simulink model "swapna_reference1"  (R2013b)
settings: Solver=ode45  StartTime=0.0  StopTime=5  RelTol=1e-3
undefined symbols (not defined in the file): sigbuilder_block, Ts_Power
libraries: powerlib x25, powerlib_meascontrol x2
settings Model: Creator=dhamodharan  LastModifiedBy=Adroit
settings DebuggingCC: StateNameClashWarn=warning

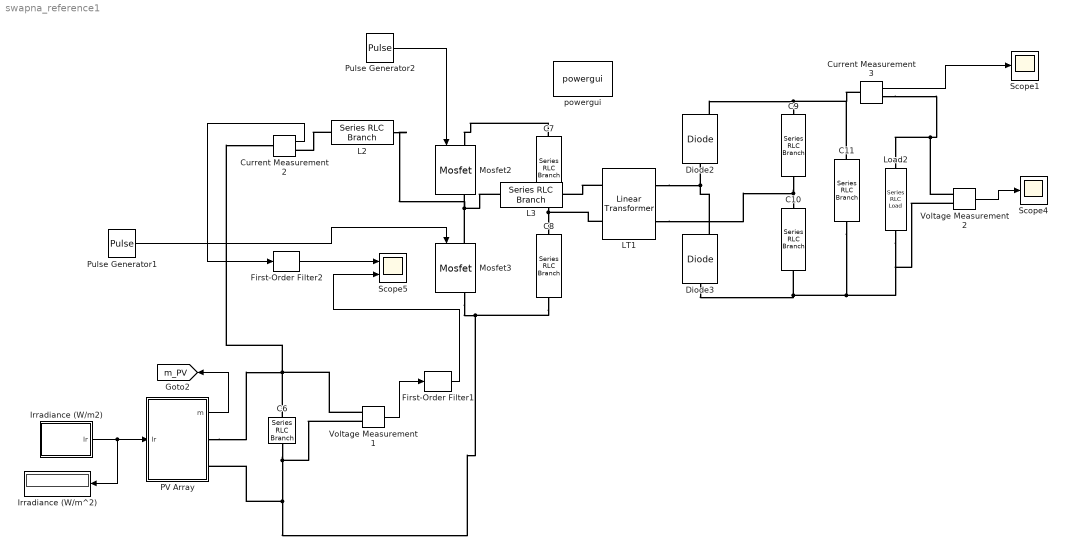
== system swapna_reference1 ==
  C10 : powerlib/Elements/Series RLC Branch  LConnTagsString=__new0  RConnTagsString=__new0  BranchType=C  Resistance=1  Inductance=1e-3  SetiL0=off  InitialCurrent=0  Capacitance=100e-9  Setx0=off  InitialVoltage=0  Measurements=None
  C11 : powerlib/Elements/Series RLC Branch  LConnTagsString=__new0  RConnTagsString=__new0  BranchType=C  Resistance=1  Inductance=1e-3  SetiL0=off  InitialCurrent=0  Capacitance=2000e-6  Setx0=off  InitialVoltage=0  Measurements=None
  C6 : powerlib/Elements/Series RLC Branch  LConnTagsString=__new0  RConnTagsString=__new0  BranchType=C  Resistance=1.0  Inductance=1.0  SetiL0=off  InitialCurrent=0  Capacitance=1000e-6  Setx0=off  InitialVoltage=0  Measurements=Branch voltage
  C7 : powerlib/Elements/Series RLC Branch  LConnTagsString=__new0  RConnTagsString=__new0  BranchType=C  Resistance=1  Inductance=1e-3  SetiL0=off  InitialCurrent=0  Capacitance=10e-6  Setx0=off  InitialVoltage=0  Measurements=None
  C8 : powerlib/Elements/Series RLC Branch  LConnTagsString=__new0  RConnTagsString=__new0  BranchType=C  Resistance=1  Inductance=1e-3  SetiL0=off  InitialCurrent=0  Capacitance=10e-6  Setx0=off  InitialVoltage=0  Measurements=None
  C9 : powerlib/Elements/Series RLC Branch  LConnTagsString=__new0  RConnTagsString=__new0  BranchType=C  Resistance=1  Inductance=1e-3  SetiL0=off  InitialCurrent=0  Capacitance=100e-9  Setx0=off  InitialVoltage=0  Measurements=None
  Current Measurement2 : powerlib/Measurements/Current Measurement  PhasorSimulation=off  OutputType=Complex  PSBequivalent=0
  Current Measurement3 : powerlib/Measurements/Current Measurement  PhasorSimulation=off  OutputType=Complex  PSBequivalent=0
  Diode2 : powerlib/Power Electronics/Diode  Ron=0.001  Lon=0  Vf=0.8  IC=0  UseSnubber=off  Rs=500  Cs=250e-9  Measurements=on
  Diode3 : powerlib/Power Electronics/Diode  Ron=0.001  Lon=0  Vf=0.8  IC=0  UseSnubber=off  Rs=500  Cs=250e-9  Measurements=on
  First-Order Filter1 : powerlib_meascontrol/Filters/First-Order Filter  FilterType=Lowpass  Tc=1/10  Ts=0  Initialize=on  Vac_Init=[0, 0, 50]  Vdc_Init=0  PlotResponse=off  FreqRange="[0,  200,  1]"
  First-Order Filter2 : powerlib_meascontrol/Filters/First-Order Filter  FilterType=Lowpass  Tc=1/1  Ts=0  Initialize=on  Vac_Init=[0, 0, 50]  Vdc_Init=0  PlotResponse=off  FreqRange="[0,  200,  1]"
  "Irradiance (W/m2) " : Subsystem  Tag=STV Subsys  LoadFcn=sigbuilder_block('load');  StartFcn=sigbuilder_block('start');  StopFcn=sigbuilder_block('stop');  ClipboardFcn=sigbuilder_block('clipboard');  mask(Sigbuilder block){}
      mask help: Sigbuilder GUI
      mask init:
      | if ~strcmp(get_param(bdroot(gcbh),'SimulationStatus'),'stopped') tuvar = sigbuilder_block('maskInit'); end
      settings: CopyFcn=sigbuilder_block('copy');  DeleteFcn=sigbuilder_block('delete');  ModelCloseFcn=sigbuilder_block('modelClose');  PreSaveFcn=sigbuilder_block('preSave');  PauseFcn=sigbuilder_block('pause')  ContinueFcn=sigbuilder_block('continue')  NameChangeFcn=sigbuilder_block('namechange');  OpenFcn=sigbuilder_block('open',[6.75 6 954 505.5 ]);  CloseFcn=sigbuilder_block('close');
      mask Display: plot(0,0,100,100,[10,10,40,40,10],[80,20,20,80,80],[40,10],[50,50], [40,27,10],[65,72,56],[40,25,25,10],[28,28,43,43]);
  Irradiance (W/m^2) : Display
      settings: Format=bank  Decimation=1000
  L2 : powerlib/Elements/Series RLC Branch  LConnTagsString=__new0  RConnTagsString=__new0  BranchType=L  Resistance=1  Inductance=100e-6  SetiL0=off  InitialCurrent=0  Capacitance=1e-6  Setx0=off  InitialVoltage=0  Measurements=None
  L3 : powerlib/Elements/Series RLC Branch  LConnTagsString=__new0  RConnTagsString=__new0  BranchType=L  Resistance=1  Inductance=0.001e-6  SetiL0=off  InitialCurrent=0  Capacitance=1e-6  Setx0=off  InitialVoltage=0  Measurements=None
  LT1 : powerlib/Elements/Linear Transformer  UNITS=pu  NominalPower=[ 200 66.66e3 ]  winding1="[ 20 0.002  0.08 ]"  winding2="[ 200 0.002  0.08 ]"  ThreeWindings=off  winding3=[ 315e3 0.002 0.08 ]  RmLm=[0.2 0.2 ]  Measurements=None  DataType=off
  Load2 : powerlib/Elements/Series RLC Load  LConnTagsString=a  RConnTagsString=__new0  NominalVoltage=120  NominalFrequency=66e3  ActivePower=30  InductivePower=0  CapacitivePower=0  Setx0=off  InitialVoltage=0  SetiL0=off  InitialCurrent=0  Measurements=None
  Mosfet2 : powerlib/Power Electronics/Mosfet  Ron=0.1  Lon=0  Rd=0.01  Vfd=0  IC=0  Rs=1e5  Cs=inf  Measurements=on
  Mosfet3 : powerlib/Power Electronics/Mosfet  Ron=0.1  Lon=0  Rd=0.01  Vfd=0  IC=0  Rs=1e5  Cs=inf  Measurements=on
  PV Array : Subsystem  mask(PV array){ModuleType=Kyocera KD135GX-LP, Ncell=36, Nser=1, Npar=2, ModuleParameters=[ 22.0999  8.36955  17.7  7.62959 ], ModelParameters=[ 0.10593  142.84  2.6762e-06  8.3758  1.5 ], Ts=Ts_Power, PlotVI_module=off, PlotVI_array=off}
      mask prompts: ModuleType "Module type:"; Ncell "Number of cells per module"; Nser "Number of series-connected  modules per string"; Npar "Number of parallel strings"; ModuleParameters "Module specifications under STC  [  Voc, Isc, Vmp, Imp ]"; ModelParameters "Model parameters for 1 module [ Rs, Rp, Isat, Iph, Qd ]"; Ts "Sample time"; PlotVI_module "Display  I-V and  P-V characteritics of one module"; PlotVI_array "Display  I-V and  P-V characteritics of array"
      mask help:
      | Model a PV array
      |
      | PV array consists of Npar strings of modules connected in parallel, each string consisting of Nser modules connected in series.
      |
      | The four PV model parameters (photo-generated current Iph, diode saturation current Isat, parallel resistance Rp and  series resistance Rs) are adjuted to fit the following four module characteristics measured under standard test conditions (STC : irradiance 1000 W/m^2, cell temperature=25 deg. C) and assuming a given "diode quality factor" (Qd) for the semiconductor:
      |   Voc = open circuit voltage
      |   Isc = short-circuit current
      |   Vmp,Imp = voltage and current at maximum power point
      |
      | Select a 'Module type' and then press Apply to see module parameters.
      | Note: Module characteristics are extracted from NREL System Advisor Model.
      mask init:
      | BlockName=gcb;
      | 
      | % Solar Modules Specifications
      | %=============================
      | %
      | Type=1;
      | SolarModuleSpec(Type).Desc= 'Kyocera KD135GX-LP';
      | SolarModuleSpec(Type).nCells= 36;              % Number of cells in series
      | SolarModuleSpec(Type).Pmp= 135.044;            % Maximum power (W)
      | SolarModuleSpec(Type).Vmp= 17.7;               % Maximum power voltage (V) 
      | SolarModuleSpec(Type).Imp= 7.62959;            % Maximum power current (A)
      | SolarModuleSpec(Type).Voc= 22.0999;            % Open circuit voltage (V)
      | SolarModuleSpec(Type).Isc= 8.36955;            % Short circuit current (A)
      | SolarModuleSpec(Type).TempC_Pmp= -6.445e-001;  % Maximum power temp. coefficient (W/deg.C)
      | SolarModuleSpec(Type).TempC_Vmp= -8.200e-002;  % Maximum power voltage temp. coefficient (V/deg.C)
      | SolarModuleSpec(Type).TempC_Imp= -1.068e-003;  % Maximum power current temp. coefficient (A/deg.C
      | SolarModuleSpec(Type).TempC_Voc= -8.000e-002;  % Open circuit voltage temp. coefficient (V/deg.C)
      | SolarModuleSpec(Type).TempC_Isc= 5.022e-003;   % Short circuit current temp. coefficient (A/deg.C)
      | SolarModuleSpec(Type).Rs= 0.10593;             % Series resistance of PV model (ohms)
      | SolarModuleSpec(Type).Rp= 142.84;              % Parallel resistance of PV model (ohms)
      | SolarModuleSpec(Type).Isat= 2.6762e-006;       % Diode saturation current of PV model (A)
      | SolarModuleSpec(Type).Iph=  8.3758;            % Light-generated photo-current  of PV model (A)
      | SolarModuleSpec(Type).Qd= 1.5;                 % Diode quality factor of PV model
      | %-------------------------------------------------------------------------
      | %
      | Type=2;
      | SolarModuleSpec(Type).Desc= 'Kyocera KD205GX-LP';
      | SolarModuleSpec(Type).nCells= 54;              % Number of cells in series
      | SolarModuleSpec(Type).Pmp= 205.075;            % Maximum power (W)
      | SolarModuleSpec(Type).Vmp= 26.6;               % Maximum power voltage (V) 
      | SolarModuleSpec(Type).Imp= 7.70959;            % Maximum power current (A)
      | SolarModuleSpec(Type).Voc= 33.1999;            % Open circuit voltage (V)
      | SolarModuleSpec(Type).Isc= 8.35955;            % Short circuit current (A)
      | SolarModuleSpec(Type).TempC_Pmp= -9.770e-001;  % Maximum power temp. coefficient (W/deg.C)
      | SolarModuleSpec(Type).TempC_Vmp= -1.230e-001;  % Maximum power voltage temp. coefficient (V/deg.C)
      | SolarModuleSpec(Type).TempC_Imp= -1.079e-003;  % Maximum power current temp. coefficient (A/deg.C
      | SolarModuleSpec(Type).TempC_Voc= -1.200e-001;  % Open circuit voltage temp. coefficient (V/deg.C)
      | SolarModuleSpec(Type).TempC_Isc= 5.016e-003;   % Short circuit current temp. coefficient (A/deg.C)
      | SolarModuleSpec(Type).Rs= 0.15943;             % Series resistance of PV model (ohms)
      | SolarModuleSpec(Type).Rp= 931.61;              % Parallel resistance of PV model (ohms)
      | SolarModuleSpec(Type).Isat= 2.647e-006;        % Diode saturation current of PV model (A)
      | SolarModuleSpec(Type).Iph= 8.3652;             % Light-generated photo-current  of PV model (A)
      | SolarModuleSpec(Type).Qd= 1.5;                 % Diode quality factor of PV model
      | %-------------------------------------------------------------------------
      | %
      | Type=3;
      | SolarModuleSpec(Type).Desc= 'Mitsubishi PV-UD190MF5';
      | SolarModuleSpec(Type).nCells= 50;              % Number of cells in series
      | SolarModuleSpec(Type).Pmp= 190.503;            % Maximum power (W)
      | SolarModuleSpec(Type).Vmp= 24.6999;            % Maximum power voltage (V) 
      | SolarModuleSpec(Type).Imp= 7.71272;            % Maximum power current (A)
      | SolarModuleSpec(Type).Voc= 30.8006;            % Open circuit voltage (V)
      | SolarModuleSpec(Type).Isc= 8.23289;            % Short circuit current (A)
      | SolarModuleSpec(Type).TempC_Pmp= -8.597e-001;  % Maximum power temp. coefficient (W/deg.C)
      | SolarModuleSpec(Type).TempC_Vmp= -1.090e-001;  % Maximum power voltage temp. coefficient (V/deg.C)
      | SolarModuleSpec(Type).TempC_Imp= -7.713e-004;  % Maximum power current temp. coefficient (A/deg.C
      | SolarModuleSpec(Type).TempC_Voc= -1.050e-001;  % Open circuit voltage temp. coefficient (V/deg.C)
      | SolarModuleSpec(Type).TempC_Isc= 4.446e-003;   % Short circuit current temp. coefficient (A/deg.C)
      | SolarModuleSpec(Type).Rs= 0.14743;             % Series resistance of PV model (ohms)
      | SolarModuleSpec(Type).Rp= 1982.4;              % Parallel resistance of PV model (ohms)
      | SolarModuleSpec(Type).Isat= 2.5519e-006;       % Diode saturation current of PV model (A)
      | SolarModuleSpec(Type).Iph= 8.2998;             % Light-generated photo-current  of PV model (A)
      | SolarModuleSpec(Type).Qd= 1.5;                 % Diode quality factor of PV model
      | %-------------------------------------------------------------------------
      | %
      | Type=4;
      | SolarModuleSpec(Type).Desc= 'Sanyo HIP-225HDE1';
      | SolarModuleSpec(Type).nCells= 60;              % Number of cells in series
      | SolarModuleSpec(Type).Pmp= 224.899;            % Maximum power (W)
      | SolarModuleSpec(Type).Vmp= 33.9;               % Maximum power voltage (V) 
      | SolarModuleSpec(Type).Imp= 6.63419;            % Maximum power current (A)
      | SolarModuleSpec(Type).Voc= 41.7984;            % Open circuit voltage (V)
      | SolarModuleSpec(Type).Isc= 7.13383;            % Short circuit current (A)
      | SolarModuleSpec(Type).TempC_Pmp= -6.925e-001;  % Maximum power temp. coefficient (W/deg.C)
      | SolarModuleSpec(Type).TempC_Vmp= -1.010e-001;  % Maximum power voltage temp. coefficient (V/deg.C)
      | SolarModuleSpec(Type).TempC_Imp= -6.634e-004;  % Maximum power current temp. coefficient (A/deg.C
      | SolarModuleSpec(Type).TempC_Voc= -1.050e-001;  % Open circuit voltage temp. coefficient (V/deg.C)
      | SolarModuleSpec(Type).TempC_Isc= 2.140e-003;   % Short circuit current temp. coefficient (A/deg.C)
      | SolarModuleSpec(Type).Rs=  0.24713;            % Series resistance of PV model (ohms)
      | SolarModuleSpec(Type).Rp= 1215.2;              % Parallel resistance of PV model (ohms)
      | SolarModuleSpec(Type).Isat= 2.697e-007;        % Diode saturation current of PV model (A)
      | SolarModuleSpec(Type).Iph= 7.1361;             % Light-generated photo-current  of PV model (A)
      | SolarModuleSpec(Type).Qd= 1.5;                 % Diode quality factor of PV model
      | %-------------------------------------------------------------------------
      | %
      | Type=5;
      | % SolarModuleSpec(Type).Desc= 'SunPower SPR-305-WHT [2009]';
      | % SolarModuleSpec(Type).nCells= 96;              % Number of cells in series
      | % SolarModuleSpec(Type).Pmp= 304.248;            % Maximum power (W)
      | % SolarModuleSpec(Type).Vmp= 54.4299;            % Maximum power voltage (V) 
      | % SolarModuleSpec(Type).Imp= 5.58972;            % Maximum power current (A)
      | % SolarModuleSpec(Type).Voc= 65.3099;            % Open circuit voltage (V)
      | % SolarModuleSpec(Type).Isc= 5.9197;             % Short circuit current (A)
      | % SolarModuleSpec(Type).TempC_Pmp= -1.229e+000;  % Maximum power temp. coefficient (W/deg.C)
      | % SolarModuleSpec(Type).TempC_Vmp= -2.030e-001;  % Maximum power voltage temp. coefficient (V/deg.C)
      | % SolarModuleSpec(Type).TempC_Imp= -1.733e-003;  % Maximum power current temp. coefficient (A/deg.C
      | % SolarModuleSpec(Type).TempC_Voc= -1.930e-001;  % Open circuit voltage temp. coefficient (V/deg.C)
      | % SolarModuleSpec(Type).TempC_Isc= 2.368e-003;   % Short circuit current temp. coefficient (A/deg.C)
      | 
      | %NREL : 2007(E)
      | SolarModuleSpec(Type).Desc= 'SunPower SPR-305-WHT';
      | SolarModuleSpec(Type).nCells= 96;              % Number of cells in series
      | SolarModuleSpec(Type).Pmp= 305.2;              % Maximum power (W)
      | SolarModuleSpec(Type).Vmp= 54.70;              % Maximum power voltage (V) 
      | SolarModuleSpec(Type).Imp= 5.58;               % Maximum power current (A)
      | SolarModuleSpec(Type).Voc= 64.20;              % Open circuit voltage (V)
      | SolarModuleSpec(Type).Isc= 5.96;               % Short circuit current (A)
      | SolarModuleSpec(Type).TempC_Pmp= -1.154e+000;  % Maximum power temp. coefficient (W/deg.C)
      | SolarModuleSpec(Type).TempC_Vmp= -1.860e-001;  % Maximum power voltage temp. coefficient (V/deg.C)
      | SolarModuleSpec(Type).TempC_Imp= -2.120e-003;  % Maximum power current temp. coefficient (A/deg.C
      | SolarModuleSpec(Type).TempC_Voc= -1.770e-001;  % Open circuit voltage temp. coefficient (V/deg.C)
      | SolarModuleSpec(Type).TempC_Isc= 3.516e-003;   % Short circuit current temp. coefficient (A/deg.C)
      | SolarModuleSpec(Type).Rs= 0.0380;              % Series resistance of PV model (ohms)
      | SolarModuleSpec(Type).Rp= 993.5;               % Parallel resistance of PV model (ohms)
      | SolarModuleSpec(Type).Isat= 3.1949e-8;         % Diode saturation current of PV model (A)
      | SolarModuleSpec(Type).Iph= 5.9602;             % Light-generated photo-current  of PV model (A)
      | SolarModuleSpec(Type).Qd= 1.3;                 % Diode quality factor of PV model
      | %-------------------------------------------------------------------------
      | %
      | Type=6;
      | SolarModuleSpec(Type).Desc= 'Suntech STP270S-24_Vb';
      | SolarModuleSpec(Type).nCells= 72;              % Number of cells in series
      | SolarModuleSpec(Type).Pmp= 269.843;            % Maximum power (W)
      | SolarModuleSpec(Type).Vmp= 35;                 % Maximum power voltage (V) 
      | SolarModuleSpec(Type).Imp= 7.70979;            % Maximum power current (A)
      | SolarModuleSpec(Type).Voc= 44.4999;            % Open circuit voltage (V)
      | SolarModuleSpec(Type).Isc= 8.19978;            % Short circuit current (A)
      | SolarModuleSpec(Type).TempC_Pmp= -1.204e+000;  % Maximum power temp. coefficient (W/deg.C)
      | SolarModuleSpec(Type).TempC_Vmp= -1.567e-001;  % Maximum power voltage temp. coefficient (V/deg.C)
      | SolarModuleSpec(Type).TempC_Imp= 1.234e-004;   % Maximum power current temp. coefficient (A/deg.C
      | SolarModuleSpec(Type).TempC_Voc= -1.504e-001;  % Open circuit voltage temp. coefficient (V/deg.C)
      | SolarModuleSpec(Type).TempC_Isc= 4.969e-003;   % Short circuit current temp. coefficient (A/deg.C)
      | SolarModuleSpec(Type).Rs= 0.32042;             % Series resistance of PV model (ohms)
      | SolarModuleSpec(Type).Rp= 3363.6;              % Parallel resistance of PV model (ohms)
      | SolarModuleSpec(Type).Isat= 2.419e-006;        % Diode saturation current of PV model (A)
      | SolarModuleSpec(Type).Iph= 8.2934;             % Light-generated photo-current  of PV model (A)
      | SolarModuleSpec(Type).Qd= 1.5;                 % Diode quality factor of PV model
      | % 
      | %-------------------------------------------------------------------------
      | %
      | Type=7;
      | SolarModuleSpec(Type).Desc= 'Canadian Solar CS5P-220M';
      | SolarModuleSpec(Type).nCells= 96;              % Number of cells in series
      | SolarModuleSpec(Type).Pmp= 219.72;             % Maximum power (W)
      | SolarModuleSpec(Type).Vmp= 48.3159;            % Maximum power voltage (V) 
      | SolarModuleSpec(Type).Imp= 4.54758;            % Maximum power current (A)
      | SolarModuleSpec(Type).Voc= 59.2618;            % Open circuit voltage (V)
      | SolarModuleSpec(Type).Isc= 5.09261;            % Short circuit current (A)
      | SolarModuleSpec(Type).TempC_Pmp= -1.031e+000;  % Maximum power temp. coefficient (W/deg.C)
      | SolarModuleSpec(Type).TempC_Vmp= -2.355e-001;  % Maximum power voltage temp. coefficient (V/deg.C)
      | SolarModuleSpec(Type).TempC_Imp= 8.231e-004;   % Maximum power current temp. coefficient (A/deg.C
      | SolarModuleSpec(Type).TempC_Voc= -2.170e-001;  % Open circuit voltage temp. coefficient (V/deg.C)
      | SolarModuleSpec(Type).TempC_Isc= 2.022e-003;   % Short circuit current temp. coefficient (A/deg.C)
      | SolarModuleSpec(Type).Rs= 0.24806;             % Series resistance of PV model (ohms)
      | SolarModuleSpec(Type).Rp= 235.76;              % Parallel resistance of PV model (ohms)
      | SolarModuleSpec(Type).Isat= 1.4435e-006;       % Diode saturation current of PV model (A)
      | SolarModuleSpec(Type).Iph= 5.098;              % Light-generated photo-current  of PV model (A)
      | SolarModuleSpec(Type).Qd= 1.5;                 % Diode quality factor of PV model
      | %-------------------------------------------------------------------------
      | %
      | Type=8;
      | SolarModuleSpec(Type).Desc= 'BP Solar SX3190';
      | SolarModuleSpec(Type).nCells= 50;              % Number of cells in series
      | SolarModuleSpec(Type).Pmp= 190.258;            % Maximum power (W)
      | SolarModuleSpec(Type).Vmp= 24.3003;            % Maximum power voltage (V) 
      | SolarModuleSpec(Type).Imp= 7.82945;            % Maximum power current (A)
      | SolarModuleSpec(Type).Voc= 30.6021;            % Open circuit voltage (V)
      | SolarModuleSpec(Type).Isc= 8.51029;            % Short circuit current (A)
      | SolarModuleSpec(Type).TempC_Pmp= -9.306e-001;  % Maximum power temp. coefficient (W/deg.C)
      | SolarModuleSpec(Type).TempC_Vmp= -1.140e-001;  % Maximum power voltage temp. coefficient (V/deg.C)
      | SolarModuleSpec(Type).TempC_Imp= -1.566e-003;  % Maximum power current temp. coefficient (A/deg.C
      | SolarModuleSpec(Type).TempC_Voc= -1.110e-001;  % Open circuit voltage temp. coefficient (V/deg.C)
      | SolarModuleSpec(Type).TempC_Isc= 5.532e-003;   % Short circuit current temp. coefficient (A/deg.C)
      | SolarModuleSpec(Type).Rs= 0.17514;             % Series resistance of PV model (ohms)
      | SolarModuleSpec(Type).Rp= 766.69;              % Parallel resistance of PV model (ohms)
      | SolarModuleSpec(Type).Isat= 2.8943e-006;       % Diode saturation current of PV model (A)
      | SolarModuleSpec(Type).Iph= 8.5156;             % Light-generated photo-current  of PV model (A)
      | SolarModuleSpec(Type).Qd= 1.5;                 % Diode quality factor of PV model
      | %-------------------------------------------------------------------------
      | %
      | Type=9;
      | SolarModuleSpec(Type).Desc= 'First Solar FS-272';
      | SolarModuleSpec(Type).nCells= 116;             % Number of cells in series
      | SolarModuleSpec(Type).Pmp= 71.326;             % Maximum power (W)
      | SolarModuleSpec(Type).Vmp= 70.558;             % Maximum power voltage (V) 
      | SolarModuleSpec(Type).Imp= 1.01088;            % Maximum power current (A)
      | SolarModuleSpec(Type).Voc= 94.5738;            % Open circuit voltage (V)
      | SolarModuleSpec(Type).Isc= 1.18103;            % Short circuit current (A)
      | SolarModuleSpec(Type).TempC_Pmp= -2.332e-001;  % Maximum power temp. coefficient (W/deg.C)
      | SolarModuleSpec(Type).TempC_Vmp= -2.060e-001;  % Maximum power voltage temp. coefficient (V/deg.C)
      | SolarModuleSpec(Type).TempC_Imp= -3.538e-004;  % Maximum power current temp. coefficient (A/deg.C
      | SolarModuleSpec(Type).TempC_Voc= -2.690e-001;  % Open circuit voltage temp. coefficient (V/deg.C)
      | SolarModuleSpec(Type).TempC_Isc= 5.433e-004;   % Short circuit current temp. coefficient (A/deg.C)
      | SolarModuleSpec(Type).Rs= 9.1791;              % Series resistance of PV model (ohms)
      | SolarModuleSpec(Type).Rp= 877.05;              % Parallel resistance of PV model (ohms)
      | SolarModuleSpec(Type).Isat= 3.7627e-007;       % Diode saturation current of PV model (A)
      | SolarModuleSpec(Type).Iph= 1.1934;             % Light-generated photo-current  of PV model (A)
      | SolarModuleSpec(Type).Qd= 2.0;                 % Diode quality factor of PV model
      | %-------------------------------------------------------------------------
      | %
      | Type=10;
      | SolarModuleSpec(Type).Desc= 'SunPower 128-cell Module';
      | SolarModuleSpec(Type).nCells= 128;             % Number of cells in series
      | SolarModuleSpec(Type).Pmp= 400.048;            % Maximum power (W)
      | SolarModuleSpec(Type).Vmp= 72.8992;            % Maximum power voltage (V) 
      | SolarModuleSpec(Type).Imp= 5.48769;            % Maximum power current (A)
      | SolarModuleSpec(Type).Voc= 85.2983;            % Open circuit voltage (V)
      | SolarModuleSpec(Type).Isc= 5.8675;             % Short circuit current (A)
      | SolarModuleSpec(Type).TempC_Pmp= -1.638e+000;  % Maximum power temp. coefficient (W/deg.C)
      | SolarModuleSpec(Type).TempC_Vmp= -2.760e-001;  % Maximum power voltage temp. coefficient (V/deg.C)
      | SolarModuleSpec(Type).TempC_Imp= -1.690e-003;  % Maximum power current temp. coefficient (A/deg.C
      | SolarModuleSpec(Type).TempC_Voc= -2.664e-001;  % Open circuit voltage temp. coefficient (V/deg.C)
      | SolarModuleSpec(Type).TempC_Isc= 1.837e-003;   % Short circuit current temp. coefficient (A/deg.C)
      | SolarModuleSpec(Type).Rs= 0.12264;             % Series resistance of PV model (ohms)
      | SolarModuleSpec(Type).Rp= 859.93;              % Parallel resistance of PV model (ohms)
      | SolarModuleSpec(Type).Isat= 6.3567e-009;       % Diode saturation current of PV model (A)
      | SolarModuleSpec(Type).Iph= 5.8683;             % Light-generated photo-current  of PV model (A)
      | SolarModuleSpec(Type).Qd= 1.2;                 % Diode quality factor of PV model
      | %-------------------------------------------------------------------------
      | 
      | Type=strmatch(ModuleType,char(SolarModuleSpec.Desc));
      | 
      | k= 1.3806e-23; % Boltman consstant (J.K^-1)
      | q=1.6022e-19;  % electron charge  (C)
      | T=273+25;
      | 
      | nCells=SolarModuleSpec(Type).nCells;
      | Voc=SolarModuleSpec(Type).Voc;
      | Isc=SolarModuleSpec(Type).Isc;
      | Vm=SolarModuleSpec(Type).Vmp;
      | Im=SolarModuleSpec(Type).Imp;
      | 
      | set_param(BlockName,'Ncell',num2str(nCells));
      | str=sprintf('[ %g  %g  %g  %g ]',Voc,Isc,Vm,Im);
      | set_param(BlockName,'ModuleParameters',str);
      | 
      | Rs=SolarModuleSpec(Type).Rs;
      | Rp=SolarModuleSpec(Type).Rp; 
      | Isat=SolarModuleSpec(Type).Isat;
      | Iph=SolarModuleSpec(Type).Iph;            
      | Qd=SolarModuleSpec(Type).Qd;
      | 
      | VT=k*T/q*nCells*Qd;
      | 
      | str=sprintf('[ %g  %g  %g  %g  %g ]',Rs,Rp,Isat,Iph, Qd);
      | set_param(BlockName,'ModelParameters',str)
      | 
      | Iph_array=Iph*Npar;
      | Isat_array=Isat*Npar;
      | VT_array=VT*Nser;
      | Rs_array=Rs*Nser/Npar;
      | Rp_array=Rp*Nser/Npar;
      | %
      | %% Plot I-V & P-V characteristics of one module
      | %==============================================
      | if PlotVI_module | PlotVI_array
      |     assignin('base','Voc',Voc);
      |     assignin('base','Isc',Isc);
      |     assignin('base','Rs',Rs);
      |     assignin('base','Rp',Rp);
      |     assignin('base','Isat',Isat);
      |     assignin('base','VT',VT);
      |      
      |     if PlotVI_module, 
      |         F1=figure('Name','I-V and P-V characteristics of one module at 25 deg.C');
      |     end
      |     if PlotVI_array ,
      |         F2=figure('Name','I-V and P-V characteristics of array at 25 deg.C');  
      |     end
      |     load_system('PV_model_Param');
      |     
      |     for ksun=1:-0.25:0.25
      |         assignin('base','Iph',Iph*ksun)
      |         sim('PV_model_Param');
      |         n=find(I_PV>=0);
      |         I_PV=I_PV(n);
      |         V_PV=V_PV(n);
      |         P_PV=V_PV.*I_PV;
      |         
      |         if PlotVI_module
      |             figure(F1);
      |             subplot(211)
      |             if ksun==1
      |                 plot(V_PV,I_PV,'b',[0  Vm Voc], [Isc Im 0],'ro')
      |                 text(Voc/15,Isc*1.1,'1 kW/m^2')
      |                 hold on
      |                 grid
      |             else
      |                 plot(V_PV,I_PV,'--m')
      |                 text(Voc/15, Isc*(ksun+0.1) , sprintf('%g kW/m^2',ksun))
      |             end
      | 
      |             subplot(212) 
      |             if ksun==1
      |                 plot(V_PV,P_PV,'b',[0  Vm Voc], [0 Im*Vm 0],'ro')
      |                 text(Vm*1.02,Vm*Im,'1 kW/m^2')
      |                 hold on
      |                 grid
      |             else
      |                 n= find(P_PV==max(P_PV));
      |                 plot(V_PV,P_PV,'--m', V_PV(n) , P_PV(n),'mo')
      |                 text(Vm*1.02, Vm*Im*ksun, sprintf('%g kW/m^2',ksun))
      |             end
      |             subplot(211)
      |             ylabel('Current (A)')
      |             xlabel('Voltage (V)')
      |             title(sprintf('Module type: %s',SolarModuleSpec(Type).Desc))
      |             axis_xy=axis;
      |             axis_xy(4)=Isc*1.2;
      |             axis(axis_xy);
      |             
      |             subplot(212)
      |             ylabel('Power (W)')
      |             xlabel('Voltage (V)')
      |             axis_xy=axis;
      |             axis_xy(4)=Vm*Im*1.2;
      |             axis(axis_xy);
      |                   
      |             set_param(BlockName,'PlotVI_module', 'off')
      |         end
      |         
      |         if PlotVI_array
      |             figure(F2);
      |             subplot(211)
      |             if ksun==1
      |                 plot(V_PV*Nser,I_PV*Npar,'b',[0  Vm Voc]*Nser, [Isc Im 0]*Npar,'ro')
      |                 text(Voc/15*Nser,Isc*1.1*Npar,'1 kW/m^2')
      |                 hold on
      |                 grid
      |             else
      |                 plot(V_PV*Nser,I_PV*Npar,'--m')
      |                 text(Voc*Nser/15, Isc*Npar*(ksun+0.1) , sprintf('%g kW/m^2',ksun))
      |             end
      |            
      | 
      |             subplot(212)
      |             if ksun==1
      |                 plot(V_PV*Nser,P_PV*Nser*Npar,'b',[0  Vm Voc]*Nser, [0 Im*Vm 0]*Nser*Npar,'ro')
      |                 text(Vm*Nser*1.02,Vm*Im*Nser*Npar,'1 kW/m^2')
      |                 hold on
      |                 grid
      |             else
      |                 n= find(P_PV==max(P_PV));
      |                 plot(V_PV*Nser,P_PV*Nser*Npar,'--m', V_PV(n)*Nser , P_PV(n)*Nser*Npar,'mo')
      |                 text(Vm*Nser*1.02, Vm*Im*Nser*Npar*ksun, sprintf('%g kW/m^2',ksun))
      |             end 
      |             subplot(211)
      |             ylabel('Current (A)')
      |             xlabel('Voltage (V)')
      |             title(sprintf('Array type: %s; %d series modules; %d parallel strings',SolarModuleSpec(Type).Desc,Nser,Npar));
      |             axis_xy=axis;
      |             axis_xy(4)=Isc*Npar*1.2;
      |             axis(axis_xy);
      |             
      |             subplot(212)
      |             ylabel('Power (W)')
      |             xlabel('Voltage (V)')
      |             xis_xy=axis;
      |             axis_xy(4)=Vm*Im*Nser*Npar*1.2;
      |             axis(axis_xy);
      |             
      |             set_param(BlockName,'PlotVI_array', 'off')
      |         end
      |         
      |     end  
      | end
      mask TypeOptions ModuleType: BP Solar SX3190 | Canadian Solar CS5P-220M | First Solar FS-272 | Kyocera KD135GX-LP | Kyocera KD205GX-LP | Mitsubishi PV-UD190MF5 | Sanyo HIP-225HDE1 | SunPower SPR-305-WHT | SunPower SPR-400-WHT | Suntech STP270S-24_Vb
      mask Display: image(imread('panel.jpg'))
  Pulse Generator1 : DiscretePulseGenerator  PulseType=Time based  Period=15e-6  PulseWidth=33  PhaseDelay=15e-6/2
  Pulse Generator2 : DiscretePulseGenerator  PulseType=Time based  Period=15e-6  PulseWidth=33
  Scope1 : Scope
      settings: TimeRange=5  YMin=0.257752  YMax=0.25779
  Scope4 : Scope
      settings: YMin=117.58  YMax=129.956  SaveName=ScopeData4
  Scope5 : Scope  NumInputPorts=2
      settings: YMin=8.7~8.6  YMax=9.05~9.25  SaveName=ScopeData5
  Voltage Measurement1 : powerlib/Measurements/Voltage Measurement  PhasorSimulation=off  OutputType=Complex  PSBequivalent=0
  Voltage Measurement2 : powerlib/Measurements/Voltage Measurement  PhasorSimulation=off  OutputType=Complex  PSBequivalent=0
  powergui : powerlib/powergui  Priority=1  SimulationMode=Discrete  SolverType=Tustin  SampleTime=50e-7  frequency=60  SPID=off  DisableSnubberDevices=off  DisableRonSwitches=off  DisableVfSwitches=off  SwTol=0  Interpol=off  DisplayEquations=off  frequencyindice=0  Pbase=100e6  ErrMax=1e-4  Iterations=50  UnitsV=kV  UnitsW=MW  FunctionMessages=off  echomessages=off  HookPort=off  EnableUseOfTLC=off  x0status=blocks  RestoreLinks=warning  ResistiveCurrentMeasurement=off  Frange=[0:2:500]  Ylog=off  Xlog=on  ShowGrid=off  save=off  variable=ZData  ZoomFFT=off  StartTime=0.0  cycles=1  DisplayStyle=1  fundamental=60  FreqAxis=off  MaxFrequency=1000  frequencyindicesteady=1  RmsSteady=1  display=off  Ts=0  methode=off
  tag scope: m_PV=global
  wires:
  "Irradiance (W/m2) "/1(Ir) -> Irradiance (W/m^2)/1, PV Array/1(Ir)
  PV Array/1(m) -> [m_PV]
  Voltage Measurement2/1 -> Scope4/1
  First-Order Filter1/1 -> Scope5/2
  Current Measurement3/1 -> Scope1/1
  Current Measurement2/1 -> First-Order Filter2/1
  Voltage Measurement1/1 -> First-Order Filter1/1
  First-Order Filter2/1 -> Scope5/1
  Pulse Generator2/1 -> Mosfet2/1
  Pulse Generator1/1 -> Mosfet3/1
  connections:
  L3/LConn1 -- Mosfet2/RConn1 -- Mosfet3/LConn1 -- L2/RConn1
  C6/RConn1 -- Mosfet3/RConn1 -- C8/RConn1 -- PV Array/RConn2 -- Voltage Measurement1/LConn2
  LT1/LConn2 -- C7/RConn1 -- C8/LConn1
  Diode3/RConn1 -- Diode2/LConn1 -- LT1/RConn1
  LT1/RConn2 -- C10/LConn1 -- C9/RConn1
  Diode2/RConn1 -- C11/LConn1 -- Current Measurement3/LConn1 -- C9/LConn1
  Diode3/LConn1 -- C10/RConn1 -- C11/RConn1 -- Load2/RConn1 -- Voltage Measurement2/LConn2
  C6/LConn1 -- PV Array/RConn1 -- Voltage Measurement1/LConn1 -- Current Measurement2/LConn1
  C7/LConn1 -- Mosfet2/LConn1
  L2/LConn1 -- Current Measurement2/RConn1
  LT1/LConn1 -- L3/RConn1
  Voltage Measurement2/LConn1 -- Load2/LConn1 -- Current Measurement3/RConn1

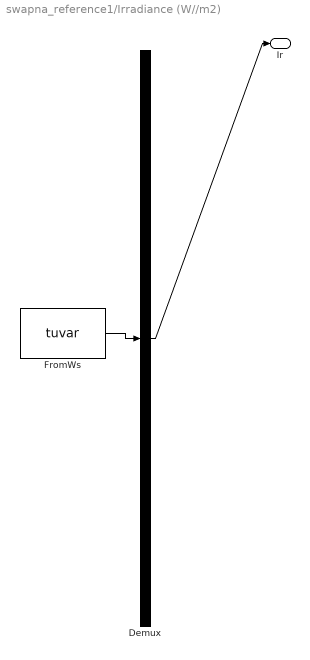
== system swapna_reference1/Irradiance (W//m2)  ==
  Demux : Demux  Tag=STV Demux  Outputs=1
  FromWs : FromWorkspace  Tag=STV FromWs  VariableName=tuvar  SampleTime=0
      SigBuilderData=|
      | common.afterFinalStr = 'Extrapolate'
      | common.sampleTime = '0'
      | dataSet(1).timeRange = [0 1]
      | dataSet(1).name = 'Constant Irradiance'
      | dataSet(2).timeRange = [0 1]
      | dataSet(2).name = 'Step Irradiance'
      | dataSet(3).timeRange = [0 3]
      | dataSet(3).name = 'Ramp-up/down Irradiance'
      | sbobj.Groups(1).Name = 'Constant Irradiance'
      | sbobj.Groups(1).Signals.Name = 'Ir'
      | sbobj.Groups(1).Signals.XData = [0 1]
      | sbobj.Groups(1).Signals.YData = [1000 1000]
      | sbobj.Groups(1).TimeRange = [0 1]
      | sbobj.Groups(2).Name = 'Step Irradiance'
      | sbobj.Groups(2).Signals.Name = 'Ir'
      | sbobj.Groups(2).Signals.XData = [0 0.501 0.51 0.69 0.7 1]
      | sbobj.Groups(2).Signals.YData = [1000 1000 250 250 1000 1000]
      | sbobj.Groups(2).TimeRange = [0 1]
      | sbobj.Groups(3).Name = 'Ramp-up/down Irradiance'
      | sbobj.Groups(3).Signals.Name = 'Ir'
      | sbobj.Groups(3).Signals.XData = [0 0.7 1.2 1.5 2 2.3 2.35 2.65 2.7 3]
      | sbobj.Groups(3).Signals.YData = [1000 1000 250 250 1000 1000 250 250 1000 1000]
      | sbobj.Groups(3).TimeRange = [0 3]
  Ir : Outport  Tag=STV Outport
  wires:
  Demux/1 -> Ir/1
  FromWs/1 -> Demux/1

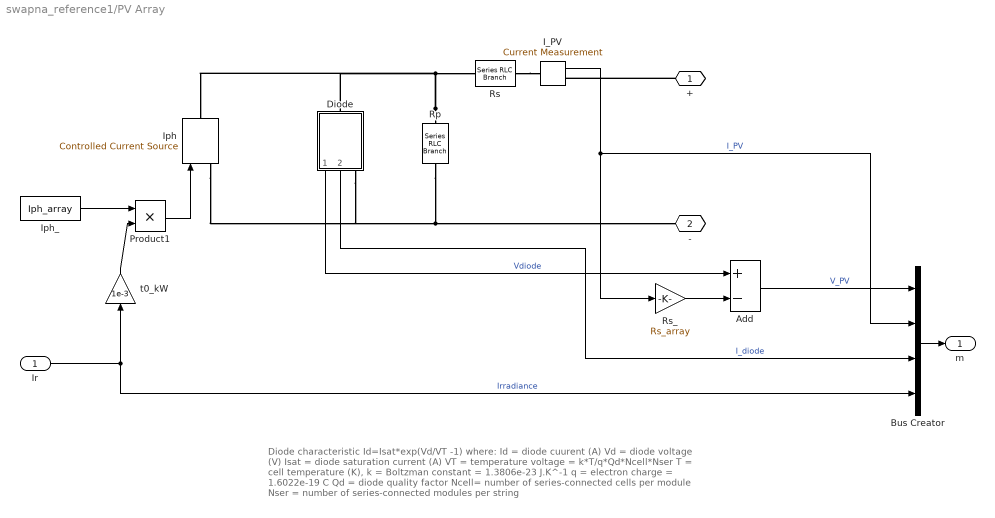
== system swapna_reference1/PV Array ==
  note: Diode characteristic
      |    Id=Isat*exp(Vd/VT -1)
      |
      | where:
      |    Id = diode cuurent (A)
      |    Vd = diode voltage (V)
      |  Isat = diode saturation current (A)
      |    VT = temperature voltage = k*T/q*Qd*Ncell*Nser
      |
      |     T = cell temperature (K),
      |     k = Boltzman constant = 1.3806e-23 J.K^-1
      |     q = electron charge = 1.6022e-19 C
      |    Qd = diode quality factor
      |  Ncell= number of series-connected cells per module
      |  Nser = number of series-connected modules per string
  Ir : Inport
  Add : Sum  Inputs=+-
  Bus Creator : BusCreator
  Diode : Subsystem
      mask Display:
      | plot(-75,-50,100,150, [-15 -15 43 -15 -15 -75],[50 8 50 92 50 50], ...
      |     [43 43],[8 94],[100 43], [50 50])
  I_PV : powerlib/Measurements/Current Measurement  PhasorSimulation=off  OutputType=Complex  PSBequivalent=0
  Iph : powerlib/Electrical Sources/Controlled Current Source  Initialize=on  Source_Type=AC  Amplitude=0  Phase=0  Frequency=0  Measurements=None
  Iph_ : Constant  Value=Iph_array
  Product1 : Product  Inputs=**  RndMeth=Zero
  Rp : powerlib/Elements/Series RLC Branch  LConnTagsString=__new0  RConnTagsString=__new0  BranchType=R  Resistance=Rp_array  Inductance=1e-3  SetiL0=off  InitialCurrent=0  Capacitance=1e-6  Setx0=off  InitialVoltage=0  Measurements=Branch current
  Rs : powerlib/Elements/Series RLC Branch  LConnTagsString=__new0  RConnTagsString=__new0  BranchType=R  Resistance=Rs_array  Inductance=1e-3  SetiL0=off  InitialCurrent=0  Capacitance=1e-6  Setx0=off  InitialVoltage=0  Measurements=None
  Rs_ : Gain  Gain=Rs_array
  t0_kW : Gain  Gain=1e-3
  + : PMIOPort  Port=1  Side=Right
  - : PMIOPort  Port=2  Side=Right
  m : Outport
  wires:
  Bus Creator/1 -> m/1
  Diode/2(Idiode) -> Bus Creator/3  "I_diode"
  Add/1 -> Bus Creator/1  "V_PV"
  t0_kW/1 -> Product1/2
  I_PV/1 -> Bus Creator/2, Rs_/1  "I_PV"
  Rs_/1 -> Add/2
  Diode/1(Vdiode) -> Add/1  "Vdiode"
  Ir/1 -> Bus Creator/4, t0_kW/1  "Irradiance"
  Iph_/1 -> Product1/1
  Product1/1 -> Iph/1
  connections:
  +/RConn1 -- I_PV/RConn1
  Rs/LConn1 -- I_PV/LConn1
  Rp/LConn1 -- Rs/RConn1 -- Iph/RConn1 -- Diode/LConn1
  Rp/RConn1 -- -/RConn1 -- Diode/RConn1 -- Iph/LConn1

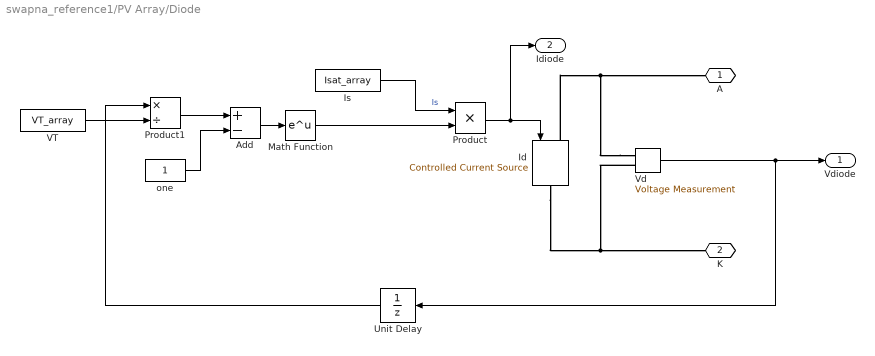
== system swapna_reference1/PV Array/Diode ==
  Add : Sum  Inputs=+-
  Id : powerlib/Electrical Sources/Controlled Current Source  Initialize=on  Source_Type=AC  Amplitude=0  Phase=0  Frequency=0  Measurements=None
  Is : Constant  Value=Isat_array
  Math Function : Math  SaturateOnIntegerOverflow=on
  Product : Product  RndMeth=Zero
  Product1 : Product  Inputs=*/  RndMeth=Zero
  Unit Delay : UnitDelay  SampleTime=Ts
  VT : Constant  Value=VT_array
  Vd : powerlib/Measurements/Voltage Measurement  PhasorSimulation=off  OutputType=Complex  PSBequivalent=0
  one : Constant
  A : PMIOPort  Port=1  Side=Left
  K : PMIOPort  Port=2  Side=Right
  Vdiode : Outport
  Idiode : Outport  Port=2
  wires:
  Product/1 -> Idiode/1, Id/1
  Vd/1 -> Vdiode/1, Unit Delay/1
  Is/1 -> Product/1  "Is"
  Product1/1 -> Add/1
  one/1 -> Add/2
  Add/1 -> Math Function/1
  Math Function/1 -> Product/2
  VT/1 -> Product1/2
  Unit Delay/1 -> Product1/1
  connections:
  Id/RConn1 -- K/RConn1 -- Vd/LConn2
  Vd/LConn1 -- A/RConn1 -- Id/LConn1
